simulink model "duffing"  (R2019b)
settings: Solver=FixedStepAuto  StartTime=0.0  StopTime=t_end  FixedStep=dt  MaxStep=.1  RelTol=1e-3
values from neighbouring files (symbols this model uses):
  beta = 1    [duffing_init.m]    (also in duffing_trim.m)
  delta = 0    [duffing_init.m]    (also in duffing_trim.m)
  gamma = 0    [duffing_init.m]    (also in duffing_trim.m)
  omega = .01    (= 0.01)    [duffing_init.m]    (also in duffing_trim.m)
  omega2 = -1    [duffing_init.m]    (also in duffing_trim.m)
  phi = 0    [duffing_init.m]    (also in duffing_trim.m)
  x0 = [0; .1]    [duffing_init.m]    (also in duffing_trim.m)
settings Model: Creator=enrique.babio  LastModifiedBy=enrique.babio
settings DataIOCC: ExternalInput=getinputstruct(opTrim)  InitialState=getstatestruct(opTrim)  LoadExternalInput=on  LoadInitialState=on  SaveState=on

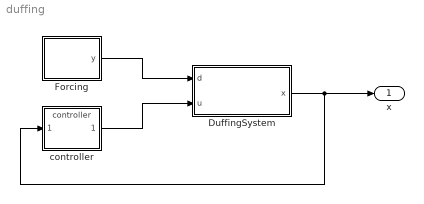
== system duffing ==
  DuffingSystem : Subsystem
  Forcing : Subsystem
  controller : ModelReference  ModelNameDialog=controller  SimulationMode=Normal  ModelReferenceVersion=1.43
  x : Outport
  wires:
  Forcing/1(y) -> DuffingSystem/1(d)
  controller/1 -> DuffingSystem/2(u)
  DuffingSystem/1(x) -> controller/1, x/1

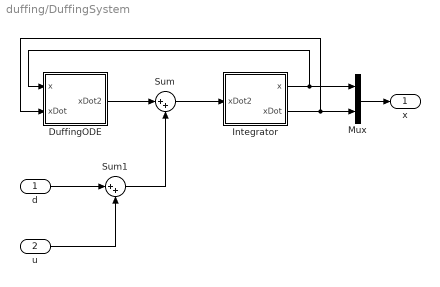
== system duffing/DuffingSystem ==
  d : Inport
  u : Inport  Port=2
  DuffingODE : Subsystem
  Integrator : Subsystem
  Mux : Mux  Inputs=2
  Sum : Sum  Inputs=|++
  Sum1 : Sum  Inputs=|++
  x : Outport
  wires:
  Integrator/1(x) -> Mux/1, DuffingODE/1(x)
  Integrator/2(xDot) -> Mux/2, DuffingODE/2(xDot)
  Mux/1 -> x/1
  DuffingODE/1(xDot2) -> Sum/1
  Sum/1 -> Integrator/1(xDot2)
  d/1 -> Sum1/1
  Sum1/1 -> Sum/2
  u/1 -> Sum1/2

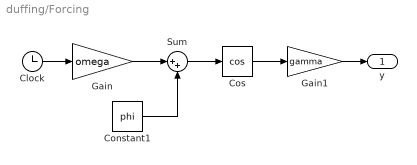
== system duffing/Forcing ==
  Clock : Clock
  Constant1 : Constant  Value=phi
  Cos : Trigonometry  Operator=cos
  Gain : Gain  Gain=omega
  Gain1 : Gain  Gain=gamma
  Sum : Sum  Inputs=|++
  y : Outport
  wires:
  Sum/1 -> Cos/1
  Clock/1 -> Gain/1
  Gain/1 -> Sum/1
  Cos/1 -> Gain1/1
  Constant1/1 -> Sum/2
  Gain1/1 -> y/1

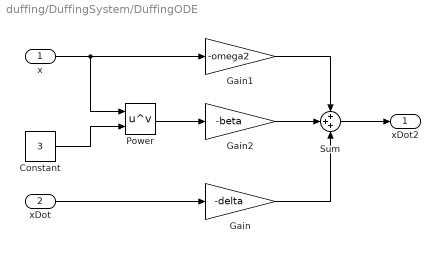
== system duffing/DuffingSystem/DuffingODE ==
  x : Inport
  xDot : Inport  Port=2
  Constant : Constant  Value=3
  Gain : Gain  Gain=-delta
  Gain1 : Gain  Gain=-omega2
  Gain2 : Gain  Gain=-beta
  Power : Math  Operator=pow  SignedPower=off  SaturateOnIntegerOverflow=on
  Sum : Sum  Inputs=+++
  xDot2 : Outport
  wires:
  x/1 -> Power/1, Gain1/1
  xDot/1 -> Gain/1
  Constant/1 -> Power/2
  Power/1 -> Gain2/1
  Sum/1 -> xDot2/1
  Gain1/1 -> Sum/1
  Gain2/1 -> Sum/2
  Gain/1 -> Sum/3

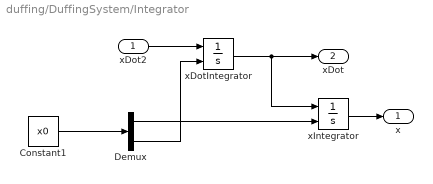
== system duffing/DuffingSystem/Integrator ==
  xDot2 : Inport
  Constant1 : Constant  Value=x0
  Demux : Demux  Outputs=2
  xDotIntegrator : Integrator  InitialConditionSource=external  InitialCondition=x0(2)  ContinuousStateAttributes='xDot'
  xIntegrator : Integrator  InitialConditionSource=external  InitialCondition=x0(1)  ZeroCross=off  ContinuousStateAttributes='x'
  x : Outport
  xDot : Outport  Port=2
  wires:
  Constant1/1 -> Demux/1
  xDotIntegrator/1 -> xDot/1, xIntegrator/1
  xDot2/1 -> xDotIntegrator/1
  xIntegrator/1 -> x/1
  Demux/1 -> xIntegrator/2
  Demux/2 -> xDotIntegrator/2
